simulink model "case4"  (R2024b)
settings: Solver=FixedStepAuto  StartTime=0  StopTime=1  FixedStep=1e-7  RelTol=1e-3
values from neighbouring files (symbols this model uses):
  SG_D_1_D = 0.01056    [IEEE9_case_parameters.m]    (also in case1_parameters.m; case2_parameters.m; case3_parameters.m; case4_parameters.m)
  SG_D_1_EnableSaturation = 0    [IEEE9_case_parameters.m]    (also in case1_parameters.m; case2_parameters.m; case3_parameters.m; case4_parameters.m)
  SG_D_1_f0 = 60    [IEEE9_case_parameters.m]    (also in case1_parameters.m; case2_parameters.m; case3_parameters.m; case4_parameters.m)
  SG_D_1_H = 7.5    [IEEE9_case_parameters.m]    (also in case1_parameters.m; case2_parameters.m; case3_parameters.m; case4_parameters.m)
  SG_D_1_K_A = 20    [IEEE9_case_parameters.m]    (also in case1_parameters.m; case2_parameters.m; case3_parameters.m; case4_parameters.m)
  SG_D_1_K_E = 1.000000e+1    (= 10)    [IEEE9_case_parameters.m]    (also in case1_parameters.m; case2_parameters.m; case3_parameters.m; case4_parameters.m)
  SG_D_1_K_F = 2.363    [IEEE9_case_parameters.m]    (also in case1_parameters.m; case2_parameters.m; case3_parameters.m; case4_parameters.m)
  SG_D_1_K_s = 0.5    [IEEE9_case_parameters.m]    (also in case1_parameters.m = 5; case2_parameters.m = 5; case3_parameters.m = 5; case4_parameters.m = 5)
  SG_D_1_R_a = 0.001088    [IEEE9_case_parameters.m]    (also in case1_parameters.m; case2_parameters.m; case3_parameters.m; case4_parameters.m)
  SG_D_1_S_A = 1    [IEEE9_case_parameters.m]    (also in case1_parameters.m; case2_parameters.m; case3_parameters.m; case4_parameters.m)
  SG_D_1_S_B = 0.103    [IEEE9_case_parameters.m]    (also in case1_parameters.m; case2_parameters.m; case3_parameters.m; case4_parameters.m)
  SG_D_1_S_N = 10.659857    [IEEE9_case_parameters.m]    (also in case1_parameters.m; case2_parameters.m; case3_parameters.m; case4_parameters.m)
  SG_D_1_SpeedPara = 200    [IEEE9_case_parameters.m]    (also in case1_parameters.m; case2_parameters.m; case3_parameters.m; case4_parameters.m)
  SG_D_1_T_0 = 0.720173    [IEEE9_case_parameters.m]    (also in case1_parameters.m = 0.755522; case2_parameters.m = 0.808931; case3_parameters.m = 0.869402; case4_parameters.m = 0.729316)
  SG_D_1_T_1 = 0.3    [IEEE9_case_parameters.m]    (also in case1_parameters.m; case2_parameters.m; case3_parameters.m; case4_parameters.m)
  SG_D_1_T_2 = 0.05    [IEEE9_case_parameters.m]    (also in case1_parameters.m; case2_parameters.m; case3_parameters.m; case4_parameters.m)
  SG_D_1_T_3 = 0.02    [IEEE9_case_parameters.m]    (also in case1_parameters.m; case2_parameters.m; case3_parameters.m; case4_parameters.m)
  SG_D_1_T_4 = 0.005    [IEEE9_case_parameters.m]    (also in case1_parameters.m; case2_parameters.m; case3_parameters.m; case4_parameters.m)
  SG_D_1_T_A = 0.02    [IEEE9_case_parameters.m]    (also in case1_parameters.m; case2_parameters.m; case3_parameters.m; case4_parameters.m)
  SG_D_1_T_dd = 8.000000e+0    (= 8)    [IEEE9_case_parameters.m]    (also in case1_parameters.m; case2_parameters.m; case3_parameters.m; case4_parameters.m)
  SG_D_1_T_ddd = 0.04    [IEEE9_case_parameters.m]    (also in case1_parameters.m; case2_parameters.m; case3_parameters.m; case4_parameters.m)
  SG_D_1_T_E = 0.314    [IEEE9_case_parameters.m]    (also in case1_parameters.m; case2_parameters.m; case3_parameters.m; case4_parameters.m)
  SG_D_1_T_F = 0.35    [IEEE9_case_parameters.m]    (also in case1_parameters.m; case2_parameters.m; case3_parameters.m; case4_parameters.m)
  SG_D_1_T_qd = 0.8    [IEEE9_case_parameters.m]    (also in case1_parameters.m; case2_parameters.m; case3_parameters.m; case4_parameters.m)
  SG_D_1_T_qdd = 0.02    [IEEE9_case_parameters.m]    (also in case1_parameters.m; case2_parameters.m; case3_parameters.m; case4_parameters.m)
  SG_D_1_T_speed = 0.1    [IEEE9_case_parameters.m]    (also in case1_parameters.m = 200; case2_parameters.m = 200; case3_parameters.m = 200; case4_parameters.m = 200)
  SG_D_1_T_w = 0.5    [IEEE9_case_parameters.m]    (also in case1_parameters.m; case2_parameters.m; case3_parameters.m; case4_parameters.m)
  SG_D_1_V_ref = 1.990276    [IEEE9_case_parameters.m]    (also in case1_parameters.m = 2.042296; case2_parameters.m = 2.051388; case3_parameters.m = 2.089584; case4_parameters.m = 2.01845)
  SG_D_1_w_ref = 376.991118    [IEEE9_case_parameters.m]    (also in case1_parameters.m; case2_parameters.m; case3_parameters.m; case4_parameters.m)
  SG_D_1_wb = 6.000000e+1    (= 60)    [IEEE9_case_parameters.m]    (also in case1_parameters.m; case2_parameters.m; case3_parameters.m; case4_parameters.m)
  SG_D_1_x_d = 1.9    [IEEE9_case_parameters.m]    (also in case1_parameters.m; case2_parameters.m; case3_parameters.m; case4_parameters.m)
  SG_D_1_x_dd = 0.302    [IEEE9_case_parameters.m]    (also in case1_parameters.m; case2_parameters.m; case3_parameters.m; case4_parameters.m)
  SG_D_1_x_ddd = 0.204    [IEEE9_case_parameters.m]    (also in case1_parameters.m; case2_parameters.m; case3_parameters.m; case4_parameters.m)
  SG_D_1_x_l = 0.05    [IEEE9_case_parameters.m]    (also in case1_parameters.m; case2_parameters.m; case3_parameters.m; case4_parameters.m)
  SG_D_1_x_q = 1.3    [IEEE9_case_parameters.m]    (also in case1_parameters.m; case2_parameters.m; case3_parameters.m; case4_parameters.m)
  SG_D_1_x_qd = 0.5    [IEEE9_case_parameters.m]    (also in case1_parameters.m; case2_parameters.m; case3_parameters.m; case4_parameters.m)
  SG_D_1_x_qdd = 0.3    [IEEE9_case_parameters.m]    (also in case1_parameters.m; case2_parameters.m; case3_parameters.m; case4_parameters.m)
  SG_D_2_D = 0.02    [IEEE9_case_parameters.m]    (also in case1_parameters.m; case2_parameters.m; case3_parameters.m; case4_parameters.m)
  SG_D_2_EnableSaturation = 0    [IEEE9_case_parameters.m]    (also in case1_parameters.m; case2_parameters.m; case3_parameters.m; case4_parameters.m)
  SG_D_2_f0 = 60    [IEEE9_case_parameters.m]    (also in case1_parameters.m; case2_parameters.m; case3_parameters.m; case4_parameters.m)
  SG_D_2_H = 8.000000e+0    (= 8)    [IEEE9_case_parameters.m]    (also in case1_parameters.m; case2_parameters.m; case3_parameters.m; case4_parameters.m)
  SG_D_2_K_A = 20    [IEEE9_case_parameters.m]    (also in case1_parameters.m; case2_parameters.m; case3_parameters.m; case4_parameters.m)
  SG_D_2_K_E = 1.000000e+1    (= 10)    [IEEE9_case_parameters.m]    (also in case1_parameters.m; case2_parameters.m; case3_parameters.m; case4_parameters.m)
  SG_D_2_K_F = 2.363    [IEEE9_case_parameters.m]    (also in case1_parameters.m; case2_parameters.m; case3_parameters.m; case4_parameters.m)
  SG_D_2_K_s = 0.5    [IEEE9_case_parameters.m]    (also in case1_parameters.m = 4; case2_parameters.m = 4; case3_parameters.m = 4; case4_parameters.m = 4)
  SG_D_2_R_a = 0.001088    [IEEE9_case_parameters.m]    (also in case1_parameters.m; case2_parameters.m; case3_parameters.m; case4_parameters.m)
  SG_D_2_S_A = 1    [IEEE9_case_parameters.m]    (also in case1_parameters.m; case2_parameters.m; case3_parameters.m; case4_parameters.m)
  SG_D_2_S_B = 0.103    [IEEE9_case_parameters.m]    (also in case1_parameters.m; case2_parameters.m; case3_parameters.m; case4_parameters.m)
  SG_D_2_S_N = 10.659857    [IEEE9_case_parameters.m]    (also in case1_parameters.m; case2_parameters.m; case3_parameters.m; case4_parameters.m)
  SG_D_2_SpeedPara = 200    [IEEE9_case_parameters.m]    (also in case1_parameters.m; case2_parameters.m; case3_parameters.m; case4_parameters.m)
  SG_D_2_T_0 = 1.632913    [IEEE9_case_parameters.m]    (also in case1_parameters.m = 1.632925; case2_parameters.m = 1.632915; case3_parameters.m = 1.632914; case4_parameters.m = 1.632927)
  SG_D_2_T_1 = 0.2    [IEEE9_case_parameters.m]    (also in case1_parameters.m; case2_parameters.m; case3_parameters.m; case4_parameters.m)
  SG_D_2_T_2 = 0.05    [IEEE9_case_parameters.m]    (also in case1_parameters.m; case2_parameters.m; case3_parameters.m; case4_parameters.m)
  SG_D_2_T_3 = 0.02    [IEEE9_case_parameters.m]    (also in case1_parameters.m; case2_parameters.m; case3_parameters.m; case4_parameters.m)
  SG_D_2_T_4 = 0.005    [IEEE9_case_parameters.m]    (also in case1_parameters.m; case2_parameters.m; case3_parameters.m; case4_parameters.m)
  SG_D_2_T_A = 0.02    [IEEE9_case_parameters.m]    (also in case1_parameters.m; case2_parameters.m; case3_parameters.m; case4_parameters.m)
  SG_D_2_T_dd = 7.9    [IEEE9_case_parameters.m]    (also in case1_parameters.m; case2_parameters.m; case3_parameters.m; case4_parameters.m)
  SG_D_2_T_ddd = 0.04    [IEEE9_case_parameters.m]    (also in case1_parameters.m; case2_parameters.m; case3_parameters.m; case4_parameters.m)
  SG_D_2_T_E = 0.314    [IEEE9_case_parameters.m]    (also in case1_parameters.m; case2_parameters.m; case3_parameters.m; case4_parameters.m)
  SG_D_2_T_F = 0.35    [IEEE9_case_parameters.m]    (also in case1_parameters.m; case2_parameters.m; case3_parameters.m; case4_parameters.m)
  SG_D_2_T_qd = 0.8    [IEEE9_case_parameters.m]    (also in case1_parameters.m; case2_parameters.m; case3_parameters.m; case4_parameters.m)
  SG_D_2_T_qdd = 0.015    [IEEE9_case_parameters.m]    (also in case1_parameters.m; case2_parameters.m; case3_parameters.m; case4_parameters.m)
  SG_D_2_T_speed = 0.1    [IEEE9_case_parameters.m]    (also in case1_parameters.m = 150; case2_parameters.m = 150; case3_parameters.m = 150; case4_parameters.m = 150)
  SG_D_2_T_w = 0.35    [IEEE9_case_parameters.m]    (also in case1_parameters.m; case2_parameters.m; case3_parameters.m; case4_parameters.m)
  SG_D_2_V_ref = 2.58547    [IEEE9_case_parameters.m]    (also in case1_parameters.m = 2.597896; case2_parameters.m = 2.587136; case3_parameters.m = 2.586042; case4_parameters.m = 2.599679)
  SG_D_2_w_ref = 376.991118    [IEEE9_case_parameters.m]    (also in case1_parameters.m; case2_parameters.m; case3_parameters.m; case4_parameters.m)
  SG_D_2_wb = 6.000000e+1    (= 60)    [IEEE9_case_parameters.m]    (also in case1_parameters.m; case2_parameters.m; case3_parameters.m; case4_parameters.m)
  SG_D_2_x_d = 1.8    [IEEE9_case_parameters.m]    (also in case1_parameters.m; case2_parameters.m; case3_parameters.m; case4_parameters.m)
  SG_D_2_x_dd = 0.302    [IEEE9_case_parameters.m]    (also in case1_parameters.m; case2_parameters.m; case3_parameters.m; case4_parameters.m)
  SG_D_2_x_ddd = 0.204    [IEEE9_case_parameters.m]    (also in case1_parameters.m; case2_parameters.m; case3_parameters.m; case4_parameters.m)
  SG_D_2_x_l = 0.05    [IEEE9_case_parameters.m]    (also in case1_parameters.m; case2_parameters.m; case3_parameters.m; case4_parameters.m)
  SG_D_2_x_q = 1.25    [IEEE9_case_parameters.m]    (also in case1_parameters.m; case2_parameters.m; case3_parameters.m; case4_parameters.m)
  SG_D_2_x_qd = 0.5    [IEEE9_case_parameters.m]    (also in case1_parameters.m; case2_parameters.m; case3_parameters.m; case4_parameters.m)
  SG_D_2_x_qdd = 0.3    [IEEE9_case_parameters.m]    (also in case1_parameters.m; case2_parameters.m; case3_parameters.m; case4_parameters.m)
  SG_D_3_D = 0.02    [IEEE9_case_parameters.m]    (also in case1_parameters.m; case2_parameters.m; case3_parameters.m; case4_parameters.m)
  SG_D_3_EnableSaturation = 0    [IEEE9_case_parameters.m]    (also in case1_parameters.m; case2_parameters.m; case3_parameters.m; case4_parameters.m)
  SG_D_3_f0 = 60    [IEEE9_case_parameters.m]    (also in case1_parameters.m; case2_parameters.m; case3_parameters.m; case4_parameters.m)
  SG_D_3_H = 7.7    [IEEE9_case_parameters.m]    (also in case1_parameters.m; case2_parameters.m; case3_parameters.m; case4_parameters.m)
  SG_D_3_K_A = 20    [IEEE9_case_parameters.m]    (also in case1_parameters.m; case2_parameters.m; case3_parameters.m; case4_parameters.m)
  SG_D_3_K_E = 1.000000e+1    (= 10)    [IEEE9_case_parameters.m]    (also in case1_parameters.m; case2_parameters.m; case3_parameters.m; case4_parameters.m)
  SG_D_3_K_F = 2.363    [IEEE9_case_parameters.m]    (also in case1_parameters.m; case2_parameters.m; case3_parameters.m; case4_parameters.m)
  SG_D_3_K_s = 0.2    [IEEE9_case_parameters.m]    (also in case1_parameters.m = 2; case2_parameters.m = 2; case3_parameters.m = 2; case4_parameters.m = 2)
  SG_D_3_R_a = 0.001088    [IEEE9_case_parameters.m]    (also in case1_parameters.m; case2_parameters.m; case3_parameters.m; case4_parameters.m)
  SG_D_3_S_A = 1    [IEEE9_case_parameters.m]    (also in case1_parameters.m; case2_parameters.m; case3_parameters.m; case4_parameters.m)
  SG_D_3_S_B = 0.103    [IEEE9_case_parameters.m]    (also in case1_parameters.m; case2_parameters.m; case3_parameters.m; case4_parameters.m)
  SG_D_3_S_N = 10.659857    [IEEE9_case_parameters.m]    (also in case1_parameters.m; case2_parameters.m; case3_parameters.m; case4_parameters.m)
  SG_D_3_SpeedPara = 200    [IEEE9_case_parameters.m]    (also in case1_parameters.m; case2_parameters.m; case3_parameters.m; case4_parameters.m)
  SG_D_3_T_0 = 0.850788    [IEEE9_case_parameters.m]    (also in case1_parameters.m = 0.850786; case2_parameters.m = 0.850787; case3_parameters.m; case4_parameters.m = 0.850786)
  SG_D_3_T_1 = 0.2    [IEEE9_case_parameters.m]    (also in case1_parameters.m; case2_parameters.m; case3_parameters.m; case4_parameters.m)
  SG_D_3_T_2 = 0.05    [IEEE9_case_parameters.m]    (also in case1_parameters.m; case2_parameters.m; case3_parameters.m; case4_parameters.m)
  SG_D_3_T_3 = 0.02    [IEEE9_case_parameters.m]    (also in case1_parameters.m; case2_parameters.m; case3_parameters.m; case4_parameters.m)
  SG_D_3_T_4 = 0.005    [IEEE9_case_parameters.m]    (also in case1_parameters.m; case2_parameters.m; case3_parameters.m; case4_parameters.m)
  SG_D_3_T_A = 0.02    [IEEE9_case_parameters.m]    (also in case1_parameters.m; case2_parameters.m; case3_parameters.m; case4_parameters.m)
  SG_D_3_T_dd = 8.1    [IEEE9_case_parameters.m]    (also in case1_parameters.m; case2_parameters.m; case3_parameters.m; case4_parameters.m)
  SG_D_3_T_ddd = 0.04    [IEEE9_case_parameters.m]    (also in case1_parameters.m; case2_parameters.m; case3_parameters.m; case4_parameters.m)
  SG_D_3_T_E = 0.314    [IEEE9_case_parameters.m]    (also in case1_parameters.m; case2_parameters.m; case3_parameters.m; case4_parameters.m)
  SG_D_3_T_F = 0.35    [IEEE9_case_parameters.m]    (also in case1_parameters.m; case2_parameters.m; case3_parameters.m; case4_parameters.m)
  SG_D_3_T_qd = 0.8    [IEEE9_case_parameters.m]    (also in case1_parameters.m; case2_parameters.m; case3_parameters.m; case4_parameters.m)
  SG_D_3_T_qdd = 0.015    [IEEE9_case_parameters.m]    (also in case1_parameters.m; case2_parameters.m; case3_parameters.m; case4_parameters.m)
  SG_D_3_T_speed = 0.1    [IEEE9_case_parameters.m]    (also in case1_parameters.m = 180; case2_parameters.m = 180; case3_parameters.m = 180; case4_parameters.m = 180)
  SG_D_3_T_w = 0.4    [IEEE9_case_parameters.m]    (also in case1_parameters.m; case2_parameters.m; case3_parameters.m; case4_parameters.m)
  SG_D_3_V_ref = 1.892727    [IEEE9_case_parameters.m]    (also in case1_parameters.m = 1.906439; case2_parameters.m = 1.895535; case3_parameters.m = 1.892105; case4_parameters.m = 1.906598)
  SG_D_3_w_ref = 376.991118    [IEEE9_case_parameters.m]    (also in case1_parameters.m; case2_parameters.m; case3_parameters.m; case4_parameters.m)
  SG_D_3_wb = 6.000000e+1    (= 60)    [IEEE9_case_parameters.m]    (also in case1_parameters.m; case2_parameters.m; case3_parameters.m; case4_parameters.m)
  SG_D_3_x_d = 1.85    [IEEE9_case_parameters.m]    (also in case1_parameters.m; case2_parameters.m; case3_parameters.m; case4_parameters.m)
  SG_D_3_x_dd = 0.302    [IEEE9_case_parameters.m]    (also in case1_parameters.m; case2_parameters.m; case3_parameters.m; case4_parameters.m)
  SG_D_3_x_ddd = 0.204    [IEEE9_case_parameters.m]    (also in case1_parameters.m; case2_parameters.m; case3_parameters.m; case4_parameters.m)
  SG_D_3_x_l = 0.05    [IEEE9_case_parameters.m]    (also in case1_parameters.m; case2_parameters.m; case3_parameters.m; case4_parameters.m)
  SG_D_3_x_q = 1.2    [IEEE9_case_parameters.m]    (also in case1_parameters.m; case2_parameters.m; case3_parameters.m; case4_parameters.m)
  SG_D_3_x_qd = 0.5    [IEEE9_case_parameters.m]    (also in case1_parameters.m; case2_parameters.m; case3_parameters.m; case4_parameters.m)
  SG_D_3_x_qdd = 0.3    [IEEE9_case_parameters.m]    (also in case1_parameters.m; case2_parameters.m; case3_parameters.m; case4_parameters.m)
(part 9 of 12)

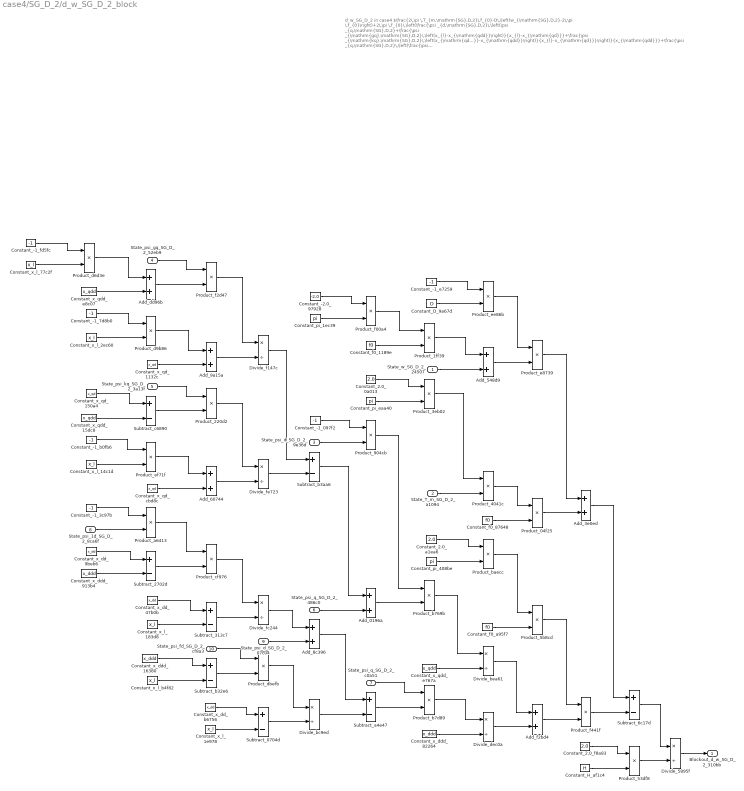
== system case4/SG_D_2/d_w_SG_D_2_block ==
  note: d_w_SG_D_2 in case4
      | $\frac{2\,\pi \,T_{m,\mathrm{SG},D,2}\,f_{0}-D\,\left(w_{\mathrm{SG},D,2}-2\,\pi \,f_{0}\right)+2\,\pi \,f_{0}\,\left(\frac{\psi _{d,\mathrm{SG},D,2}\,\left(\psi _{q,\mathrm{SG},D,2}+\frac{\psi _{\mathrm{gq},\mathrm{SG},D,2}\,\left(x_{l}-x_{\mathrm{qdd}}\right)}{x_{l}-x_{\mathrm{qd}}}+\frac{\psi _{\mathrm{kq},\mathrm{SG},D,2}\,\left(x_{\mathrm{qd}}-x_{\mathrm{qdd}}\right)}{x_{l}-x_{\mathrm{qd}}}\right)}{x_{\mathrm{qdd}}}+\frac{\psi _{q,\mathrm{SG},D,2}\,\left(\frac{\psi _{\mathrm{1d},\mathrm{SG},D,2}\,\left(x_{\mathrm{dd}}-x_{\mathrm{ddd}}\right)}{x_{\mathrm{dd}}-x_{l}}-\psi _{d,\mathrm{SG},D,2}+\frac{\psi _{\mathrm{fd},\mathrm{SG},D,2}\,\left(x_{\mathrm{ddd}}-x_{l}\right)}{x_{\mathrm{dd}}-x_{l}}\right)}{x_{\mathrm{ddd}}}\right)}{2\,H}$
      | Automatically generated on 2025-10-31 19:05:37 .
  State_w_SG_D_2_24507 : Inport
  State_T_m_SG_D_2_a1094 : Inport  Port=2
  State_psi_d_SG_D_2_9e36d : Inport  Port=3
  State_psi_gq_SG_D_2_52eb9 : Inport  Port=4
  State_psi_kq_SG_D_2_3a13f : Inport  Port=5
  State_psi_q_SG_D_2_486c0 : Inport  Port=6
  State_psi_q_SG_D_2_c0a51 : Inport  Port=7
  State_psi_1d_SG_D_2_8ca6f : Inport  Port=8
  State_psi_d_SG_D_2_07c04 : Inport  Port=9
  State_psi_fd_SG_D_2_cf8a3 : Inport  Port=10
  Add_0196a : Sum
  Add_3e0ed : Sum
  Add_548d9 : Sum
  Add_60744 : Sum
  Add_8c396 : Sum
  Add_9a15a : Sum
  Add_dd96b : Sum
  Add_f2bd4 : Sum
  Constant_-1_097f2 : Constant  Value=-1
  Constant_-1_3c97b : Constant  Value=-1
  Constant_-1_7d8b0 : Constant  Value=-1
  Constant_-1_b0fb6 : Constant  Value=-1
  Constant_-1_e7259 : Constant  Value=-1
  Constant_-1_fd5fc : Constant  Value=-1
  Constant_-2.0_97928 : Constant  Value=-2.0
  Constant_2.0_0a013 : Constant  Value=2.0
  Constant_2.0_a1ea6 : Constant  Value=2.0
  Constant_2.0_f8a83 : Constant  Value=2.0
  Constant_D_9a67d : Constant  Value=D
  Constant_H_af1c4 : Constant  Value=H
  Constant_f0_1189e : Constant  Value=f0
  Constant_f0_87648 : Constant  Value=f0
  Constant_f0_a95f7 : Constant  Value=f0
  Constant_pi_1ec39 : Constant  Value=pi
  Constant_pi_408be : Constant  Value=pi
  Constant_pi_eaa40 : Constant  Value=pi
  Constant_x_dd_47b0b : Constant  Value=x_dd
  Constant_x_dd_9beb6 : Constant  Value=x_dd
  Constant_x_dd_b6756 : Constant  Value=x_dd
  Constant_x_ddd_16380 : Constant  Value=x_ddd
  Constant_x_ddd_82264 : Constant  Value=x_ddd
  Constant_x_ddd_913b4 : Constant  Value=x_ddd
  Constant_x_l_14c1d : Constant  Value=x_l
  Constant_x_l_183d8 : Constant  Value=x_l
  Constant_x_l_1e978 : Constant  Value=x_l
  Constant_x_l_2ec60 : Constant  Value=x_l
  Constant_x_l_77c2f : Constant  Value=x_l
  Constant_x_l_b4f82 : Constant  Value=x_l
  Constant_x_qd_1132c : Constant  Value=x_qd
  Constant_x_qd_150a4 : Constant  Value=x_qd
  Constant_x_qd_cbd8c : Constant  Value=x_qd
  Constant_x_qdd_15dc8 : Constant  Value=x_qdd
  Constant_x_qdd_e767a : Constant  Value=x_qdd
  Constant_x_qdd_e8c07 : Constant  Value=x_qdd
  Divide_5895f : Product  Inputs=*/
  Divide_bc9ed : Product  Inputs=*/
  Divide_bea61 : Product  Inputs=*/
  Divide_dec0a : Product  Inputs=*/
  Divide_f147c : Product  Inputs=*/
  Divide_fc244 : Product  Inputs=*/
  Divide_fe723 : Product  Inputs=*/
  Product_04f25 : Product
  Product_1ff39 : Product
  Product_220d2 : Product
  Product_3eb02 : Product
  Product_4041c : Product
  Product_53df8 : Product
  Product_5b8cd : Product
  Product_904cb : Product
  Product_a6413 : Product
  Product_b769b : Product
  Product_b7d89 : Product
  Product_baecc : Product
  Product_cf976 : Product
  Product_d6d3e : Product
  Product_d9b86 : Product
  Product_dbefb : Product
  Product_e8739 : Product
  Product_ee86b : Product
  Product_ef71f : Product
  Product_f00a4 : Product
  Product_f2d47 : Product
  Product_f441f : Product
  Subtract_0704d : Sum  Inputs=+-
  Subtract_2702d : Sum  Inputs=+-
  Subtract_313c7 : Sum  Inputs=+-
  Subtract_6c17d : Sum  Inputs=+-
  Subtract_a4e47 : Sum  Inputs=+-
  Subtract_b32e6 : Sum  Inputs=+-
  Subtract_b3aa6 : Sum  Inputs=+-
  Subtract_c6890 : Sum  Inputs=+-
  Blockout_d_w_SG_D_2_310bb : Outport
  wires:
  Constant_x_qd_150a4/1 -> Subtract_c6890/1
  Constant_-1_b0fb6/1 -> Product_ef71f/1
  Constant_-1_fd5fc/1 -> Product_d6d3e/1
  Constant_x_qdd_15dc8/1 -> Subtract_c6890/2
  Subtract_0704d/1 -> Divide_bc9ed/2
  Constant_x_l_14c1d/1 -> Product_ef71f/2
  Constant_x_l_77c2f/1 -> Product_d6d3e/2
  Product_ef71f/1 -> Add_60744/1
  Product_d6d3e/1 -> Add_dd96b/1
  Constant_x_l_183d8/1 -> Subtract_313c7/2
  Constant_x_l_2ec60/1 -> Product_d9b86/2
  Constant_x_ddd_82264/1 -> Divide_dec0a/2
  Subtract_b32e6/1 -> Product_dbefb/2
  Constant_x_qd_cbd8c/1 -> Add_60744/2
  Constant_x_qdd_e8c07/1 -> Add_dd96b/2
  Constant_-1_7d8b0/1 -> Product_d9b86/1
  State_psi_d_SG_D_2_9e36d/1 -> Product_904cb/2
  Constant_-1_3c97b/1 -> Product_a6413/1
  State_w_SG_D_2_24507/1 -> Add_548d9/2
  Product_d9b86/1 -> Add_9a15a/1
  State_psi_1d_SG_D_2_8ca6f/1 -> Product_a6413/2
  Constant_x_dd_9beb6/1 -> Subtract_2702d/1
  Divide_f147c/1 -> Subtract_b3aa6/1
  Subtract_c6890/1 -> Product_220d2/2
  Constant_x_ddd_913b4/1 -> Subtract_2702d/2
  State_psi_gq_SG_D_2_52eb9/1 -> Product_f2d47/1
  Add_60744/1 -> Divide_fe723/2
  State_psi_d_SG_D_2_07c04/1 -> Add_8c396/2
  Add_dd96b/1 -> Product_f2d47/2
  Constant_x_qd_1132c/1 -> Add_9a15a/2
  State_psi_kq_SG_D_2_3a13f/1 -> Product_220d2/1
  Product_a6413/1 -> Product_cf976/1
  Subtract_2702d/1 -> Product_cf976/2
  Constant_pi_eaa40/1 -> Product_3eb02/2
  Constant_x_dd_47b0b/1 -> Subtract_313c7/1
  Constant_x_ddd_16380/1 -> Subtract_b32e6/1
  Constant_x_l_b4f82/1 -> Subtract_b32e6/2
  Product_f2d47/1 -> Divide_f147c/1
  Add_9a15a/1 -> Divide_f147c/2
  Add_0196a/1 -> Product_b769b/2
  Product_220d2/1 -> Divide_fe723/1
  Constant_pi_1ec39/1 -> Product_f00a4/2
  Product_cf976/1 -> Divide_fc244/1
  Subtract_313c7/1 -> Divide_fc244/2
  State_psi_fd_SG_D_2_cf8a3/1 -> Product_dbefb/1
  Divide_fc244/1 -> Add_8c396/1
  Constant_x_dd_b6756/1 -> Subtract_0704d/1
  Constant_x_l_1e978/1 -> Subtract_0704d/2
  Divide_fe723/1 -> Subtract_b3aa6/2
  Product_dbefb/1 -> Divide_bc9ed/1
  Constant_-1_097f2/1 -> Product_904cb/1
  Constant_-2.0_97928/1 -> Product_f00a4/1
  Subtract_b3aa6/1 -> Add_0196a/1
  Subtract_a4e47/1 -> Product_b7d89/2
  State_psi_q_SG_D_2_486c0/1 -> Add_0196a/2
  Constant_D_9a67d/1 -> Product_ee86b/2
  Add_8c396/1 -> Subtract_a4e47/1
  Divide_bc9ed/1 -> Subtract_a4e47/2
  Product_f00a4/1 -> Product_1ff39/1
  Constant_f0_1189e/1 -> Product_1ff39/2
  Constant_2.0_0a013/1 -> Product_3eb02/1
  Product_904cb/1 -> Product_b769b/1
  State_psi_q_SG_D_2_c0a51/1 -> Product_b7d89/1
  Constant_-1_e7259/1 -> Product_ee86b/1
  Product_1ff39/1 -> Add_548d9/1
  Product_3eb02/1 -> Product_4041c/1
  State_T_m_SG_D_2_a1094/1 -> Product_4041c/2
  Constant_2.0_a1ea6/1 -> Product_baecc/1
  Constant_pi_408be/1 -> Product_baecc/2
  Product_b769b/1 -> Divide_bea61/1
  Constant_x_qdd_e767a/1 -> Divide_bea61/2
  Product_b7d89/1 -> Divide_dec0a/1
  Product_ee86b/1 -> Product_e8739/1
  Add_548d9/1 -> Product_e8739/2
  Product_4041c/1 -> Product_04f25/1
  Constant_f0_87648/1 -> Product_04f25/2
  Product_baecc/1 -> Product_5b8cd/1
  Constant_f0_a95f7/1 -> Product_5b8cd/2
  Divide_bea61/1 -> Add_f2bd4/1
  Divide_dec0a/1 -> Add_f2bd4/2
  Product_e8739/1 -> Add_3e0ed/1
  Product_04f25/1 -> Add_3e0ed/2
  Product_5b8cd/1 -> Product_f441f/1
  Add_f2bd4/1 -> Product_f441f/2
  Add_3e0ed/1 -> Subtract_6c17d/1
  Product_f441f/1 -> Subtract_6c17d/2
  Constant_2.0_f8a83/1 -> Product_53df8/1
  Constant_H_af1c4/1 -> Product_53df8/2
  Subtract_6c17d/1 -> Divide_5895f/1
  Product_53df8/1 -> Divide_5895f/2
  Divide_5895f/1 -> Blockout_d_w_SG_D_2_310bb/1

== system case4/SG_D_2/i_d_SG_D_2_block ==
  note: i_d_SG_D_2 in case4
      | $\frac{\sin\left(\theta _{\mathrm{SG},D,2}\right)\,\left(\frac{\psi _{\mathrm{1d},\mathrm{SG},D,2}\,\left(x_{\mathrm{dd}}-x_{\mathrm{ddd}}\right)}{x_{\mathrm{dd}}-x_{l}}-\psi _{d,\mathrm{SG},D,2}+\frac{\psi _{\mathrm{fd},\mathrm{SG},D,2}\,\left(x_{\mathrm{ddd}}-x_{l}\right)}{x_{\mathrm{dd}}-x_{l}}\right)}{x_{\mathrm{ddd}}}-\frac{\cos\left(\theta _{\mathrm{SG},D,2}\right)\,\left(\psi _{q,\mathrm{SG},D,2}+\frac{\psi _{\mathrm{gq},\mathrm{SG},D,2}\,\left(x_{l}-x_{\mathrm{qdd}}\right)}{x_{l}-x_{\mathrm{qd}}}+\frac{\psi _{\mathrm{kq},\mathrm{SG},D,2}\,\left(x_{\mathrm{qd}}-x_{\mathrm{qdd}}\right)}{x_{l}-x_{\mathrm{qd}}}\right)}{x_{\mathrm{qdd}}}$
      | Automatically generated on 2025-10-31 19:05:57 .
  State_psi_gq_SG_D_2_b50ef : Inport
  State_psi_kq_SG_D_2_4dc54 : Inport  Port=2
  State_psi_q_SG_D_2_d9bdd : Inport  Port=3
  State_theta_SG_D_2_d89e5 : Inport  Port=4
  State_psi_1d_SG_D_2_5ca32 : Inport  Port=5
  State_psi_d_SG_D_2_cc06c : Inport  Port=6
  State_psi_fd_SG_D_2_3594a : Inport  Port=7
  State_theta_SG_D_2_c3678 : Inport  Port=8
  Add_2bfec : Sum
  Add_4eafa : Sum
  Add_6bd05 : Sum
  Add_7f92b : Sum
  Add_e5599 : Sum
  Constant_-1_2a19b : Constant  Value=-1
  Constant_-1_314f4 : Constant  Value=-1
  Constant_-1_6f956 : Constant  Value=-1
  Constant_-1_74ab8 : Constant  Value=-1
  Constant_-1_7d589 : Constant  Value=-1
  Constant_x_dd_1112f : Constant  Value=x_dd
  Constant_x_dd_28043 : Constant  Value=x_dd
  Constant_x_dd_93079 : Constant  Value=x_dd
  Constant_x_ddd_14e97 : Constant  Value=x_ddd
  Constant_x_ddd_53be7 : Constant  Value=x_ddd
  Constant_x_ddd_a4ee9 : Constant  Value=x_ddd
  Constant_x_l_09ea4 : Constant  Value=x_l
  Constant_x_l_125c2 : Constant  Value=x_l
  Constant_x_l_97056 : Constant  Value=x_l
  Constant_x_l_d3fa2 : Constant  Value=x_l
  Constant_x_l_f09d9 : Constant  Value=x_l
  Constant_x_l_f7cfa : Constant  Value=x_l
  Constant_x_qd_08ada : Constant  Value=x_qd
  Constant_x_qd_50310 : Constant  Value=x_qd
  Constant_x_qd_b6060 : Constant  Value=x_qd
  Constant_x_qdd_1d7d4 : Constant  Value=x_qdd
  Constant_x_qdd_8d76d : Constant  Value=x_qdd
  Constant_x_qdd_bcb21 : Constant  Value=x_qdd
  Divide_1e09e : Product  Inputs=*/
  Divide_518a4 : Product  Inputs=*/
  Divide_bc6c1 : Product  Inputs=*/
  Divide_cd719 : Product  Inputs=*/
  Divide_d2eaf : Product  Inputs=*/
  Divide_ec618 : Product  Inputs=*/
  MathFunc_cos_8af24 : Trigonometry  Operator=cos
  MathFunc_sin_6591e : Trigonometry
  Product_17c2a : Product
  Product_36218 : Product
  Product_3c1c4 : Product
  Product_53a98 : Product
  Product_6191f : Product
  Product_64df0 : Product
  Product_a2cae : Product
  Product_a4238 : Product
  Product_b9b1d : Product
  Product_c1e9b : Product
  Product_da60c : Product
  Subtract_21e43 : Sum  Inputs=+-
  Subtract_2b410 : Sum  Inputs=+-
  Subtract_3e074 : Sum  Inputs=+-
  Subtract_46cbf : Sum  Inputs=+-
  Subtract_86df4 : Sum  Inputs=+-
  Subtract_caeb0 : Sum  Inputs=+-
  Subtract_cba65 : Sum  Inputs=+-
  Subtract_fb917 : Sum  Inputs=+-
  Blockout_i_d_SG_D_2_51594 : Outport
  wires:
  Constant_x_ddd_53be7/1 -> Subtract_46cbf/1
  Constant_x_qd_50310/1 -> Subtract_86df4/1
  Constant_-1_7d589/1 -> Product_17c2a/1
  Constant_-1_314f4/1 -> Product_53a98/1
  Subtract_21e43/1 -> Blockout_i_d_SG_D_2_51594/1
  Constant_x_qdd_bcb21/1 -> Subtract_86df4/2
  Constant_x_l_f09d9/1 -> Product_17c2a/2
  Constant_x_l_d3fa2/1 -> Product_53a98/2
  Product_17c2a/1 -> Add_6bd05/1
  Product_53a98/1 -> Add_7f92b/1
  Constant_x_l_f7cfa/1 -> Product_36218/2
  Constant_x_qd_b6060/1 -> Add_6bd05/2
  Constant_x_qdd_1d7d4/1 -> Add_7f92b/2
  Constant_x_qdd_8d76d/1 -> Divide_bc6c1/2
  MathFunc_cos_8af24/1 -> Product_b9b1d/2
  Constant_-1_74ab8/1 -> Product_36218/1
  State_psi_gq_SG_D_2_b50ef/1 -> Product_6191f/1
  Subtract_46cbf/1 -> Product_c1e9b/2
  Product_64df0/1 -> Product_3c1c4/1
  Add_6bd05/1 -> Divide_518a4/2
  Add_7f92b/1 -> Product_6191f/2
  Product_c1e9b/1 -> Divide_ec618/1
  Product_36218/1 -> Add_4eafa/1
  Constant_x_qd_08ada/1 -> Add_4eafa/2
  State_theta_SG_D_2_c3678/1 -> MathFunc_sin_6591e/1
  State_psi_kq_SG_D_2_4dc54/1 -> Product_a4238/1
  Add_2bfec/1 -> Subtract_2b410/1
  Subtract_86df4/1 -> Product_a4238/2
  Product_6191f/1 -> Divide_cd719/1
  Constant_-1_6f956/1 -> Product_64df0/1
  State_psi_1d_SG_D_2_5ca32/1 -> Product_64df0/2
  State_psi_fd_SG_D_2_3594a/1 -> Product_c1e9b/1
  Constant_x_dd_28043/1 -> Subtract_3e074/1
  Product_3c1c4/1 -> Divide_1e09e/1
  Constant_x_ddd_14e97/1 -> Subtract_3e074/2
  Divide_ec618/1 -> Subtract_2b410/2
  Add_4eafa/1 -> Divide_cd719/2
  Product_da60c/1 -> Divide_d2eaf/1
  Product_a4238/1 -> Divide_518a4/1
  Constant_-1_2a19b/1 -> Product_a2cae/1
  Subtract_fb917/1 -> Divide_ec618/2
  Subtract_3e074/1 -> Product_3c1c4/2
  Constant_x_dd_1112f/1 -> Subtract_caeb0/1
  Subtract_2b410/1 -> Product_da60c/1
  Constant_x_l_09ea4/1 -> Subtract_caeb0/2
  Constant_x_l_97056/1 -> Subtract_46cbf/2
  Divide_cd719/1 -> Subtract_cba65/1
  Divide_d2eaf/1 -> Subtract_21e43/2
  Divide_518a4/1 -> Subtract_cba65/2
  Subtract_caeb0/1 -> Divide_1e09e/2
  Constant_x_dd_93079/1 -> Subtract_fb917/1
  Divide_bc6c1/1 -> Subtract_21e43/1
  Constant_x_l_125c2/1 -> Subtract_fb917/2
  Subtract_cba65/1 -> Add_e5599/1
  State_psi_q_SG_D_2_d9bdd/1 -> Add_e5599/2
  Constant_x_ddd_a4ee9/1 -> Divide_d2eaf/2
  MathFunc_sin_6591e/1 -> Product_da60c/2
  Divide_1e09e/1 -> Add_2bfec/1
  State_psi_d_SG_D_2_cc06c/1 -> Add_2bfec/2
  Add_e5599/1 -> Product_a2cae/2
  State_theta_SG_D_2_d89e5/1 -> MathFunc_cos_8af24/1
  Product_a2cae/1 -> Product_b9b1d/1
  Product_b9b1d/1 -> Divide_bc6c1/1

== system case4/SG_D_2/i_q_SG_D_2_block ==
  note: i_q_SG_D_2 in case4
      | $-\frac{\sin\left(\theta _{\mathrm{SG},D,2}\right)\,\left(\psi _{q,\mathrm{SG},D,2}+\frac{\psi _{\mathrm{gq},\mathrm{SG},D,2}\,\left(x_{l}-x_{\mathrm{qdd}}\right)}{x_{l}-x_{\mathrm{qd}}}+\frac{\psi _{\mathrm{kq},\mathrm{SG},D,2}\,\left(x_{\mathrm{qd}}-x_{\mathrm{qdd}}\right)}{x_{l}-x_{\mathrm{qd}}}\right)}{x_{\mathrm{qdd}}}-\frac{\cos\left(\theta _{\mathrm{SG},D,2}\right)\,\left(\frac{\psi _{\mathrm{1d},\mathrm{SG},D,2}\,\left(x_{\mathrm{dd}}-x_{\mathrm{ddd}}\right)}{x_{\mathrm{dd}}-x_{l}}-\psi _{d,\mathrm{SG},D,2}+\frac{\psi _{\mathrm{fd},\mathrm{SG},D,2}\,\left(x_{\mathrm{ddd}}-x_{l}\right)}{x_{\mathrm{dd}}-x_{l}}\right)}{x_{\mathrm{ddd}}}$
      | Automatically generated on 2025-10-31 19:06:01 .
  State_psi_gq_SG_D_2_b06e0 : Inport
  State_psi_kq_SG_D_2_4278f : Inport  Port=2
  State_psi_q_SG_D_2_089b8 : Inport  Port=3
  State_theta_SG_D_2_9d528 : Inport  Port=4
  State_psi_1d_SG_D_2_35b9d : Inport  Port=5
  State_psi_d_SG_D_2_1475e : Inport  Port=6
  State_psi_fd_SG_D_2_02c56 : Inport  Port=7
  State_theta_SG_D_2_f85ec : Inport  Port=8
  Add_23aa0 : Sum
  Add_477b5 : Sum
  Add_53ec0 : Sum
  Add_a659a : Sum
  Add_dddda : Sum
  Add_efb3a : Sum
  Constant_-1_198e1 : Constant  Value=-1
  Constant_-1_548c7 : Constant  Value=-1
  Constant_-1_5778c : Constant  Value=-1
  Constant_-1_5ae42 : Constant  Value=-1
  Constant_-1_f4a6f : Constant  Value=-1
  Constant_x_dd_1549f : Constant  Value=x_dd
  Constant_x_dd_4fc62 : Constant  Value=x_dd
  Constant_x_dd_5e42b : Constant  Value=x_dd
  Constant_x_ddd_092a7 : Constant  Value=x_ddd
  Constant_x_ddd_0e071 : Constant  Value=x_ddd
  Constant_x_ddd_5f668 : Constant  Value=x_ddd
  Constant_x_l_14401 : Constant  Value=x_l
  Constant_x_l_29c47 : Constant  Value=x_l
  Constant_x_l_70fdc : Constant  Value=x_l
  Constant_x_l_78ff8 : Constant  Value=x_l
  Constant_x_l_7b18b : Constant  Value=x_l
  Constant_x_l_978fc : Constant  Value=x_l
  Constant_x_qd_0efda : Constant  Value=x_qd
  Constant_x_qd_935a1 : Constant  Value=x_qd
  Constant_x_qd_e3dc8 : Constant  Value=x_qd
  Constant_x_qdd_15b64 : Constant  Value=x_qdd
  Constant_x_qdd_93812 : Constant  Value=x_qdd
  Constant_x_qdd_a509b : Constant  Value=x_qdd
  Divide_0c0b4 : Product  Inputs=*/
  Divide_3be6b : Product  Inputs=*/
  Divide_57fc1 : Product  Inputs=*/
  Divide_667bc : Product  Inputs=*/
  Divide_7cfe4 : Product  Inputs=*/
  Divide_f2708 : Product  Inputs=*/
  MathFunc_cos_87c9e : Trigonometry  Operator=cos
  MathFunc_sin_2077c : Trigonometry
  Product_20b04 : Product
  Product_2425a : Product
  Product_4eed3 : Product
  Product_58854 : Product
  Product_7e356 : Product
  Product_9dcb9 : Product
  Product_a3c58 : Product
  Product_b7c6d : Product
  Product_e346e : Product
  Product_e78a5 : Product
  Product_f7b98 : Product
  Subtract_141d3 : Sum  Inputs=+-
  Subtract_3c09a : Sum  Inputs=+-
  Subtract_4b073 : Sum  Inputs=+-
  Subtract_707a4 : Sum  Inputs=+-
  Subtract_9f90e : Sum  Inputs=+-
  Subtract_cb979 : Sum  Inputs=+-
  Subtract_d34ea : Sum  Inputs=+-
  Blockout_i_q_SG_D_2_f7c08 : Outport
  wires:
  MathFunc_sin_2077c/1 -> Product_e346e/2
  Product_b7c6d/1 -> Product_e346e/1
  Constant_-1_548c7/1 -> Product_20b04/1
  Constant_-1_198e1/1 -> Product_e78a5/1
  Constant_x_l_7b18b/1 -> Product_20b04/2
  Product_20b04/1 -> Add_23aa0/1
  Subtract_cb979/1 -> Product_58854/2
  Constant_x_qdd_93812/1 -> Subtract_141d3/2
  Constant_x_qdd_15b64/1 -> Add_23aa0/2
  Add_a659a/1 -> Product_b7c6d/2
  Constant_x_l_978fc/1 -> Product_e78a5/2
  Constant_x_qd_e3dc8/1 -> Subtract_141d3/1
  Constant_-1_5ae42/1 -> Product_a3c58/1
  Constant_x_l_29c47/1 -> Product_a3c58/2
  State_psi_1d_SG_D_2_35b9d/1 -> Product_9dcb9/2
  State_psi_gq_SG_D_2_b06e0/1 -> Product_4eed3/1
  Add_23aa0/1 -> Product_4eed3/2
  Product_e78a5/1 -> Add_477b5/1
  Divide_3be6b/1 -> Add_53ec0/1
  Constant_x_qd_935a1/1 -> Add_477b5/2
  State_psi_kq_SG_D_2_4278f/1 -> Product_7e356/1
  Add_dddda/1 -> Subtract_4b073/1
  Constant_x_ddd_5f668/1 -> Subtract_cb979/2
  Subtract_141d3/1 -> Product_7e356/2
  Product_a3c58/1 -> Add_efb3a/1
  Constant_x_qd_0efda/1 -> Add_efb3a/2
  Constant_-1_f4a6f/1 -> Product_9dcb9/1
  Constant_x_l_70fdc/1 -> Subtract_707a4/2
  Constant_x_dd_5e42b/1 -> Subtract_cb979/1
  Product_4eed3/1 -> Divide_667bc/1
  Divide_7cfe4/1 -> Subtract_4b073/2
  Add_477b5/1 -> Divide_667bc/2
  Product_2425a/1 -> Divide_f2708/1
  Product_7e356/1 -> Divide_0c0b4/1
  Constant_-1_5778c/1 -> Product_b7c6d/1
  Product_9dcb9/1 -> Product_58854/1
  Add_efb3a/1 -> Divide_0c0b4/2
  Constant_x_dd_4fc62/1 -> Subtract_9f90e/1
  Subtract_4b073/1 -> Product_2425a/1
  Subtract_d34ea/1 -> Product_f7b98/2
  Constant_x_l_14401/1 -> Subtract_9f90e/2
  Constant_x_ddd_0e071/1 -> Subtract_d34ea/1
  Constant_x_l_78ff8/1 -> Subtract_d34ea/2
  Divide_667bc/1 -> Subtract_3c09a/1
  Divide_f2708/1 -> Add_53ec0/2
  Product_f7b98/1 -> Divide_7cfe4/1
  Divide_0c0b4/1 -> Subtract_3c09a/2
  Subtract_707a4/1 -> Divide_7cfe4/2
  Product_58854/1 -> Divide_57fc1/1
  Subtract_9f90e/1 -> Divide_57fc1/2
  Constant_x_qdd_a509b/1 -> Divide_3be6b/2
  State_psi_fd_SG_D_2_02c56/1 -> Product_f7b98/1
  Constant_x_dd_1549f/1 -> Subtract_707a4/1
  Subtract_3c09a/1 -> Add_a659a/1
  State_psi_q_SG_D_2_089b8/1 -> Add_a659a/2
  Constant_x_ddd_092a7/1 -> Divide_f2708/2
  Divide_57fc1/1 -> Add_dddda/1
  State_psi_d_SG_D_2_1475e/1 -> Add_dddda/2
  State_theta_SG_D_2_9d528/1 -> MathFunc_sin_2077c/1
  State_theta_SG_D_2_f85ec/1 -> MathFunc_cos_87c9e/1
  MathFunc_cos_87c9e/1 -> Product_2425a/2
  Product_e346e/1 -> Divide_3be6b/1
  Add_53ec0/1 -> Blockout_i_q_SG_D_2_f7c08/1

== system case4/SG_D_2/theta_SG_D_2_out_block ==
  note: theta_SG_D_2_out in case4
      | $\theta _{\mathrm{SG},D,2}$
      | Automatically generated on 2025-10-31 19:06:06 .
  State_theta_SG_D_2_ce1d4 : Inport
  Blockout_theta_SG_D_2_out_e80c4 : Outport
  wires:
  State_theta_SG_D_2_ce1d4/1 -> Blockout_theta_SG_D_2_out_e80c4/1

== system case4/SG_D_2/w_SG_D_2_out_block ==
  note: w_SG_D_2_out in case4
      | $w_{\mathrm{SG},D,2}$
      | Automatically generated on 2025-10-31 19:06:05 .
  State_w_SG_D_2_49837 : Inport
  Blockout_w_SG_D_2_out_2aeb7 : Outport
  wires:
  State_w_SG_D_2_49837/1 -> Blockout_w_SG_D_2_out_2aeb7/1

== system case4/SG_D_3/T_e_SG_D_3_block ==
  note: T_e_SG_D_3 in case4
      | $-\frac{\psi _{d,\mathrm{SG},D,3}\,\left(\psi _{q,\mathrm{SG},D,3}+\frac{\psi _{\mathrm{gq},\mathrm{SG},D,3}\,\left(x_{l}-x_{\mathrm{qdd}}\right)}{x_{l}-x_{\mathrm{qd}}}+\frac{\psi _{\mathrm{kq},\mathrm{SG},D,3}\,\left(x_{\mathrm{qd}}-x_{\mathrm{qdd}}\right)}{x_{l}-x_{\mathrm{qd}}}\right)}{x_{\mathrm{qdd}}}-\frac{\psi _{q,\mathrm{SG},D,3}\,\left(\frac{\psi _{\mathrm{1d},\mathrm{SG},D,3}\,\left(x_{\mathrm{dd}}-x_{\mathrm{ddd}}\right)}{x_{\mathrm{dd}}-x_{l}}-\psi _{d,\mathrm{SG},D,3}+\frac{\psi _{\mathrm{fd},\mathrm{SG},D,3}\,\left(x_{\mathrm{ddd}}-x_{l}\right)}{x_{\mathrm{dd}}-x_{l}}\right)}{x_{\mathrm{ddd}}}$
      | Automatically generated on 2025-10-31 19:07:10 .
  State_psi_d_SG_D_3_77ae3 : Inport
  State_psi_gq_SG_D_3_d6484 : Inport  Port=2
  State_psi_kq_SG_D_3_5a7ef : Inport  Port=3
  State_psi_q_SG_D_3_b778b : Inport  Port=4
  State_psi_q_SG_D_3_ce48a : Inport  Port=5
  State_psi_1d_SG_D_3_88fd6 : Inport  Port=6
  State_psi_d_SG_D_3_80976 : Inport  Port=7
  State_psi_fd_SG_D_3_9b24b : Inport  Port=8
  Add_3851c : Sum
  Add_41a7d : Sum
  Add_55f49 : Sum
  Add_938fe : Sum
  Add_b0066 : Sum
  Add_f3fc2 : Sum
  Constant_-1_30855 : Constant  Value=-1
  Constant_-1_3bc3d : Constant  Value=-1
  Constant_-1_5a0bb : Constant  Value=-1
  Constant_-1_cce15 : Constant  Value=-1
  Constant_-1_e8aec : Constant  Value=-1
  Constant_x_dd_02b3c : Constant  Value=x_dd
  Constant_x_dd_6ffa5 : Constant  Value=x_dd
  Constant_x_dd_9a360 : Constant  Value=x_dd
  Constant_x_ddd_0ed9f : Constant  Value=x_ddd
  Constant_x_ddd_52ead : Constant  Value=x_ddd
  Constant_x_ddd_9fe87 : Constant  Value=x_ddd
  Constant_x_l_3ae3e : Constant  Value=x_l
  Constant_x_l_501e1 : Constant  Value=x_l
  Constant_x_l_7595d : Constant  Value=x_l
  Constant_x_l_85717 : Constant  Value=x_l
  Constant_x_l_a5736 : Constant  Value=x_l
  Constant_x_l_f0edd : Constant  Value=x_l
  Constant_x_qd_7f6e6 : Constant  Value=x_qd
  Constant_x_qd_80484 : Constant  Value=x_qd
  Constant_x_qd_93305 : Constant  Value=x_qd
  Constant_x_qdd_54890 : Constant  Value=x_qdd
  Constant_x_qdd_5a7a1 : Constant  Value=x_qdd
  Constant_x_qdd_badf3 : Constant  Value=x_qdd
  Divide_08935 : Product  Inputs=*/
  Divide_2aa76 : Product  Inputs=*/
  Divide_341b8 : Product  Inputs=*/
  Divide_37007 : Product  Inputs=*/
  Divide_70ec3 : Product  Inputs=*/
  Divide_da930 : Product  Inputs=*/
  Product_18272 : Product
  Product_2ed9a : Product
  Product_367f7 : Product
  Product_4dfed : Product
  Product_55329 : Product
  Product_55334 : Product
  Product_9b477 : Product
  Product_ae9ae : Product
  Product_c99cf : Product
  Product_ebfa0 : Product
  Product_feaee : Product
  Subtract_2b2ac : Sum  Inputs=+-
  Subtract_441fc : Sum  Inputs=+-
  Subtract_71ff0 : Sum  Inputs=+-
  Subtract_8181d : Sum  Inputs=+-
  Subtract_c043b : Sum  Inputs=+-
  Subtract_c777d : Sum  Inputs=+-
  Subtract_ca289 : Sum  Inputs=+-
  Blockout_T_e_SG_D_3_61551 : Outport
  wires:
  State_psi_q_SG_D_3_b778b/1 -> Add_938fe/2
  Constant_-1_5a0bb/1 -> Product_367f7/1
  Subtract_2b2ac/1 -> Product_c99cf/2
  State_psi_1d_SG_D_3_88fd6/1 -> Product_4dfed/2
  Constant_-1_30855/1 -> Product_55334/1
  Constant_x_l_7595d/1 -> Product_55334/2
  Add_b0066/1 -> Subtract_2b2ac/1
  State_psi_d_SG_D_3_80976/1 -> Add_b0066/2
  Product_55334/1 -> Add_3851c/1
  Constant_x_qdd_54890/1 -> Subtract_8181d/2
  Add_938fe/1 -> Product_55329/2
  Constant_x_qdd_5a7a1/1 -> Add_3851c/2
  State_psi_q_SG_D_3_ce48a/1 -> Product_c99cf/1
  Constant_x_l_85717/1 -> Product_367f7/2
  Subtract_c043b/1 -> Divide_37007/2
  Constant_x_l_501e1/1 -> Subtract_ca289/2
  Constant_x_qd_7f6e6/1 -> Subtract_8181d/1
  Constant_-1_cce15/1 -> Product_ebfa0/1
  Subtract_441fc/1 -> Divide_2aa76/2
  Constant_x_l_a5736/1 -> Product_ebfa0/2
  Product_feaee/1 -> Divide_2aa76/1
  Constant_-1_e8aec/1 -> Product_4dfed/1
  Product_4dfed/1 -> Product_feaee/1
  Constant_x_dd_6ffa5/1 -> Subtract_c777d/1
  Constant_x_ddd_0ed9f/1 -> Subtract_c777d/2
  Add_f3fc2/1 -> Blockout_T_e_SG_D_3_61551/1
  State_psi_gq_SG_D_3_d6484/1 -> Product_9b477/1
  Product_c99cf/1 -> Divide_70ec3/1
  Add_3851c/1 -> Product_9b477/2
  State_psi_fd_SG_D_3_9b24b/1 -> Product_ae9ae/1
  Product_367f7/1 -> Add_55f49/1
  Constant_x_qd_93305/1 -> Add_55f49/2
  Constant_x_dd_02b3c/1 -> Subtract_441fc/1
  State_psi_kq_SG_D_3_5a7ef/1 -> Product_18272/1
  Constant_x_dd_9a360/1 -> Subtract_c043b/1
  Subtract_8181d/1 -> Product_18272/2
  Product_55329/1 -> Divide_341b8/1
  Product_ebfa0/1 -> Add_41a7d/1
  Add_55f49/1 -> Divide_da930/2
  Constant_x_qd_80484/1 -> Add_41a7d/2
  Subtract_c777d/1 -> Product_feaee/2
  Constant_x_l_3ae3e/1 -> Subtract_441fc/2
  Constant_x_ddd_52ead/1 -> Subtract_ca289/1
  Product_9b477/1 -> Divide_da930/1
  Product_18272/1 -> Divide_08935/1
  Add_41a7d/1 -> Divide_08935/2
  Constant_x_ddd_9fe87/1 -> Divide_70ec3/2
  Subtract_ca289/1 -> Product_ae9ae/2
  Divide_da930/1 -> Subtract_71ff0/1
  Constant_x_l_f0edd/1 -> Subtract_c043b/2
  Divide_08935/1 -> Subtract_71ff0/2
  Divide_2aa76/1 -> Add_b0066/1
  Product_ae9ae/1 -> Divide_37007/1
  Constant_-1_3bc3d/1 -> Product_2ed9a/1
  State_psi_d_SG_D_3_77ae3/1 -> Product_2ed9a/2
  Subtract_71ff0/1 -> Add_938fe/1
  Divide_37007/1 -> Subtract_2b2ac/2
  Product_2ed9a/1 -> Product_55329/1
  Constant_x_qdd_badf3/1 -> Divide_341b8/2
  Divide_341b8/1 -> Add_f3fc2/1
  Divide_70ec3/1 -> Add_f3fc2/2

== system case4/SG_D_3/d_E_fd_SG_D_3_block ==
  note: d_E_fd_SG_D_3 in case4
      | $\frac{V_{f,\mathrm{SG},D,3}-E_{\mathrm{fd},\mathrm{SG},D,3}\,K_{E}}{T_{E}}$
      | Automatically generated on 2025-10-31 19:06:54 .
  State_E_fd_SG_D_3_21366 : Inport
  State_V_f_SG_D_3_0199b : Inport  Port=2
  Add_81159 : Sum
  Constant_-1_8bdd4 : Constant  Value=-1
  Constant_K_E_40585 : Constant  Value=K_E
  Constant_T_E_821a3 : Constant  Value=T_E
  Divide_a95b3 : Product  Inputs=*/
  Product_2c942 : Product
  Product_fe9cb : Product
  Blockout_d_E_fd_SG_D_3_64aec : Outport
  wires:
  State_V_f_SG_D_3_0199b/1 -> Add_81159/2
  Constant_-1_8bdd4/1 -> Product_2c942/1
  State_E_fd_SG_D_3_21366/1 -> Product_2c942/2
  Constant_T_E_821a3/1 -> Divide_a95b3/2
  Product_2c942/1 -> Product_fe9cb/1
  Product_fe9cb/1 -> Add_81159/1
  Constant_K_E_40585/1 -> Product_fe9cb/2
  Divide_a95b3/1 -> Blockout_d_E_fd_SG_D_3_64aec/1
  Add_81159/1 -> Divide_a95b3/1

== system case4/SG_D_3/d_Px_1_SG_D_3_block ==
  note: d_Px_1_SG_D_3 in case4
      | $\frac{w_{\mathrm{SG},D,3}-2\,\pi \,f_{0}}{T_{w}}-\frac{\mathrm{Px}_{1,\mathrm{SG},D,3}}{T_{w}}$
      | Automatically generated on 2025-10-31 19:06:55 .
  State_Px_1_SG_D_3_e066f : Inport
  State_w_SG_D_3_8a56a : Inport  Port=2
  Add_e7754 : Sum
  Add_eb1d5 : Sum
  Constant_-1_4298c : Constant  Value=-1
  Constant_-2.0_77398 : Constant  Value=-2.0
  Constant_T_w_a1c5a : Constant  Value=T_w
  Constant_T_w_d89fb : Constant  Value=T_w
  Constant_f0_c684c : Constant  Value=f0
  Constant_pi_4f391 : Constant  Value=pi
  Divide_24c12 : Product  Inputs=*/
  Divide_6bd81 : Product  Inputs=*/
  Product_01dd0 : Product
  Product_9290a : Product
  Product_a2f1c : Product
  Blockout_d_Px_1_SG_D_3_e0808 : Outport
  wires:
  Constant_f0_c684c/1 -> Product_01dd0/2
  Constant_-1_4298c/1 -> Product_9290a/1
  Constant_-2.0_77398/1 -> Product_a2f1c/1
  Constant_pi_4f391/1 -> Product_a2f1c/2
  Product_a2f1c/1 -> Product_01dd0/1
  State_w_SG_D_3_8a56a/1 -> Add_eb1d5/2
  Divide_6bd81/1 -> Add_e7754/1
  State_Px_1_SG_D_3_e066f/1 -> Product_9290a/2
  Product_01dd0/1 -> Add_eb1d5/1
  Product_9290a/1 -> Divide_6bd81/1
  Constant_T_w_d89fb/1 -> Divide_6bd81/2
  Add_eb1d5/1 -> Divide_24c12/1
  Constant_T_w_a1c5a/1 -> Divide_24c12/2
  Divide_24c12/1 -> Add_e7754/2
  Add_e7754/1 -> Blockout_d_Px_1_SG_D_3_e0808/1

== system case4/SG_D_3/d_Px_2_SG_D_3_block ==
  note: d_Px_2_SG_D_3 in case4
      | $\frac{\mathrm{Px}_{1,\mathrm{SG},D,3}-T_{2}\,\left(\frac{\mathrm{Px}_{1,\mathrm{SG},D,3}}{T_{w}}-\frac{w_{\mathrm{SG},D,3}-2\,\pi \,f_{0}}{T_{w}}\right)}{T_{1}}-\frac{\mathrm{Px}_{2,\mathrm{SG},D,3}}{T_{1}}$
      | Automatically generated on 2025-10-31 19:06:56 .
  State_Px_2_SG_D_3_881a5 : Inport
  State_Px_1_SG_D_3_d6c88 : Inport  Port=2
  State_Px_1_SG_D_3_02523 : Inport  Port=3
  State_w_SG_D_3_c73de : Inport  Port=4
  Add_0f9e0 : Sum
  Add_58989 : Sum
  Add_ac894 : Sum
  Add_ccdb3 : Sum
  Constant_-1_b8511 : Constant  Value=-1
  Constant_-1_bd3d2 : Constant  Value=-1
  Constant_-2.0_9d85f : Constant  Value=-2.0
  Constant_T_1_b40be : Constant  Value=T_1
  Constant_T_1_c67a0 : Constant  Value=T_1
  Constant_T_2_52f0a : Constant  Value=T_2
  Constant_T_w_068e4 : Constant  Value=T_w
  Constant_T_w_b0b20 : Constant  Value=T_w
  Constant_f0_5fb5d : Constant  Value=f0
  Constant_pi_b49aa : Constant  Value=pi
  Divide_05c10 : Product  Inputs=*/
  Divide_7257a : Product  Inputs=*/
  Divide_860cc : Product  Inputs=*/
  Divide_9155c : Product  Inputs=*/
  Product_0d7f4 : Product
  Product_139e4 : Product
  Product_4a5c8 : Product
  Product_72b12 : Product
  Product_924f2 : Product
  Blockout_d_Px_2_SG_D_3_8eaa1 : Outport
  wires:
  State_Px_1_SG_D_3_02523/1 -> Product_72b12/2
  Constant_-2.0_9d85f/1 -> Product_924f2/1
  Constant_f0_5fb5d/1 -> Product_4a5c8/2
  Constant_pi_b49aa/1 -> Product_924f2/2
  Product_924f2/1 -> Product_4a5c8/1
  State_w_SG_D_3_c73de/1 -> Add_ac894/2
  Constant_-1_b8511/1 -> Product_72b12/1
  Product_4a5c8/1 -> Add_ac894/1
  Product_72b12/1 -> Divide_7257a/1
  Constant_T_w_b0b20/1 -> Divide_7257a/2
  Add_ac894/1 -> Divide_05c10/1
  Constant_T_w_068e4/1 -> Divide_05c10/2
  Divide_7257a/1 -> Add_0f9e0/1
  Divide_05c10/1 -> Add_0f9e0/2
  Constant_T_2_52f0a/1 -> Product_139e4/1
  Add_0f9e0/1 -> Product_139e4/2
  Constant_-1_bd3d2/1 -> Product_0d7f4/1
  Product_139e4/1 -> Add_ccdb3/2
  State_Px_2_SG_D_3_881a5/1 -> Product_0d7f4/2
  State_Px_1_SG_D_3_d6c88/1 -> Add_ccdb3/1
  Product_0d7f4/1 -> Divide_9155c/1
  Add_58989/1 -> Blockout_d_Px_2_SG_D_3_8eaa1/1
  Constant_T_1_c67a0/1 -> Divide_9155c/2
  Add_ccdb3/1 -> Divide_860cc/1
  Constant_T_1_b40be/1 -> Divide_860cc/2
  Divide_9155c/1 -> Add_58989/1
  Divide_860cc/1 -> Add_58989/2

== system case4/SG_D_3/d_Px_3_SG_D_3_block ==
  note: d_Px_3_SG_D_3 in case4
      | $\frac{\mathrm{Px}_{2,\mathrm{SG},D,3}+T_{4}\,\left(\frac{\mathrm{Px}_{1,\mathrm{SG},D,3}-T_{2}\,\left(\frac{\mathrm{Px}_{1,\mathrm{SG},D,3}}{T_{w}}-\frac{w_{\mathrm{SG},D,3}-2\,\pi \,f_{0}}{T_{w}}\right)}{T_{1}}-\frac{\mathrm{Px}_{2,\mathrm{SG},D,3}}{T_{1}}\right)}{T_{3}}-\frac{\mathrm{Px}_{3,\mathrm{SG},D,3}}{T_{3}}$
      | Automatically generated on 2025-10-31 19:06:59 .
  State_Px_3_SG_D_3_a4ed4 : Inport
  State_Px_2_SG_D_3_9dd6f : Inport  Port=2
  State_Px_2_SG_D_3_78cc5 : Inport  Port=3
  State_Px_1_SG_D_3_a976b : Inport  Port=4
  State_Px_1_SG_D_3_b1c74 : Inport  Port=5
  State_w_SG_D_3_a3743 : Inport  Port=6
  Add_2bfa9 : Sum
  Add_3dbc6 : Sum
  Add_42a99 : Sum
  Add_703d0 : Sum
  Add_ca46d : Sum
  Add_cc49c : Sum
  Constant_-1_17318 : Constant  Value=-1
  Constant_-1_2d7a4 : Constant  Value=-1
  Constant_-1_9c1ef : Constant  Value=-1
  Constant_-2.0_26b53 : Constant  Value=-2.0
  Constant_T_1_a258b : Constant  Value=T_1
  Constant_T_1_b177d : Constant  Value=T_1
  Constant_T_2_890e2 : Constant  Value=T_2
  Constant_T_3_8a485 : Constant  Value=T_3
  Constant_T_3_e6f6b : Constant  Value=T_3
  Constant_T_4_9dd70 : Constant  Value=T_4
  Constant_T_w_a32c5 : Constant  Value=T_w
  Constant_T_w_d3f13 : Constant  Value=T_w
  Constant_f0_a5365 : Constant  Value=f0
  Constant_pi_3c10d : Constant  Value=pi
  Divide_0aff2 : Product  Inputs=*/
  Divide_9d059 : Product  Inputs=*/
  Divide_aca88 : Product  Inputs=*/
  Divide_af822 : Product  Inputs=*/
  Divide_b33db : Product  Inputs=*/
  Divide_cf04e : Product  Inputs=*/
  Product_173c0 : Product
  Product_19f50 : Product
  Product_38f98 : Product
  Product_73b81 : Product
  Product_b55d6 : Product
  Product_c8511 : Product
  Product_fee53 : Product
  Blockout_d_Px_3_SG_D_3_1ad82 : Outport
  wires:
  State_Px_1_SG_D_3_b1c74/1 -> Product_19f50/2
  Constant_f0_a5365/1 -> Product_b55d6/2
  Constant_-2.0_26b53/1 -> Product_38f98/1
  Add_ca46d/1 -> Divide_b33db/1
  Constant_pi_3c10d/1 -> Product_38f98/2
  Product_38f98/1 -> Product_b55d6/1
  State_w_SG_D_3_a3743/1 -> Add_2bfa9/2
  Constant_T_w_d3f13/1 -> Divide_aca88/2
  Constant_-1_2d7a4/1 -> Product_19f50/1
  Product_b55d6/1 -> Add_2bfa9/1
  Product_19f50/1 -> Divide_aca88/1
  Add_2bfa9/1 -> Divide_cf04e/1
  Product_fee53/1 -> Divide_0aff2/1
  Constant_T_w_a32c5/1 -> Divide_cf04e/2
  Divide_aca88/1 -> Add_3dbc6/1
  Divide_cf04e/1 -> Add_3dbc6/2
  Constant_T_2_890e2/1 -> Product_73b81/1
  Add_3dbc6/1 -> Product_73b81/2
  Constant_-1_17318/1 -> Product_fee53/1
  State_Px_2_SG_D_3_78cc5/1 -> Product_fee53/2
  State_Px_1_SG_D_3_a976b/1 -> Add_ca46d/1
  Constant_T_3_8a485/1 -> Divide_9d059/2
  Product_73b81/1 -> Add_ca46d/2
  Constant_T_1_a258b/1 -> Divide_0aff2/2
  Add_42a99/1 -> Product_c8511/2
  Constant_T_1_b177d/1 -> Divide_b33db/2
  Divide_af822/1 -> Add_703d0/2
  Divide_0aff2/1 -> Add_42a99/1
  Divide_b33db/1 -> Add_42a99/2
  Constant_T_4_9dd70/1 -> Product_c8511/1
  Constant_-1_9c1ef/1 -> Product_173c0/1
  State_Px_3_SG_D_3_a4ed4/1 -> Product_173c0/2
  State_Px_2_SG_D_3_9dd6f/1 -> Add_cc49c/1
  Product_c8511/1 -> Add_cc49c/2
  Product_173c0/1 -> Divide_9d059/1
  Add_cc49c/1 -> Divide_af822/1
  Constant_T_3_e6f6b/1 -> Divide_af822/2
  Divide_9d059/1 -> Add_703d0/1
  Add_703d0/1 -> Blockout_d_Px_3_SG_D_3_1ad82/1
